simulink model "Wheel_Moments"  (R2020a)
settings: Solver=VariableStepAuto  StartTime=0.0  StopTime=10.0  RelTol=1e-3
values from neighbouring files (symbols this model uses):
  Effective_radius = 0.2    [Properties.sldd]
  Initial_omega = 75.0    [Properties.sldd]
  Wheel_inertia = 0.0205    [Properties.sldd]
undefined symbols (not defined in the file or in its folder): Spin_switch_threshold
settings Model: DataDictionary=Properties.sldd  Creator=Matthew  LastModifiedBy=Matthew
settings ModelReferenceCC: ModelReferenceMinAlgLoopOccurrences=on

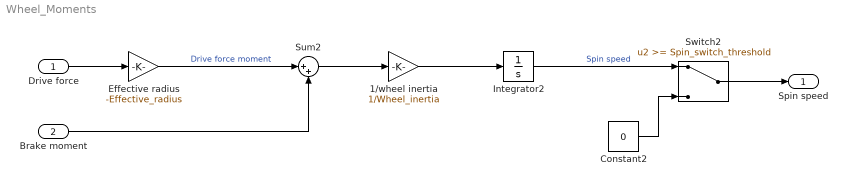
== system Wheel_Moments ==
  Drive force : Inport
  Brake moment : Inport  Port=2
  1/wheel inertia : Gain  Gain=1/Wheel_inertia
  Constant2 : Constant  Value=0
  Effective radius : Gain  Gain=-Effective_radius
  Integrator2 : Integrator  InitialCondition=Initial_omega
  Sum2 : Sum  Inputs=|++
  Switch2 : Switch  Threshold=Spin_switch_threshold
  Spin speed : Outport
  wires:
  Switch2/1 -> Spin speed/1
  Constant2/1 -> Switch2/3
  Integrator2/1 -> Switch2/1  "Spin speed"
  Sum2/1 -> 1/wheel inertia/1
  Effective radius/1 -> Sum2/1  "Drive force moment"
  Drive force/1 -> Effective radius/1
  1/wheel inertia/1 -> Integrator2/1
  Brake moment/1 -> Sum2/2
